simulink model "debugcurrentloop"  (R2024a)
settings: Solver=VariableStepAuto  StartTime=0.0  StopTime=5  RelTol=1e-3
model workspace (MAT data in the model file):
  Frequency_175 = 0
  TargetFrequency_175 = 2100000000
  uniqueStringPll_175 = '53_5733'
undefined symbols (not defined in the file): DiscIntNeverNeededParam
libraries: simulink x6, mcbcontrolslib x6, slpidlib x1, mcbplantlib x1, autolibpmsmexterior x1
settings Model: Creator=wsl  LastModifiedBy=wsl

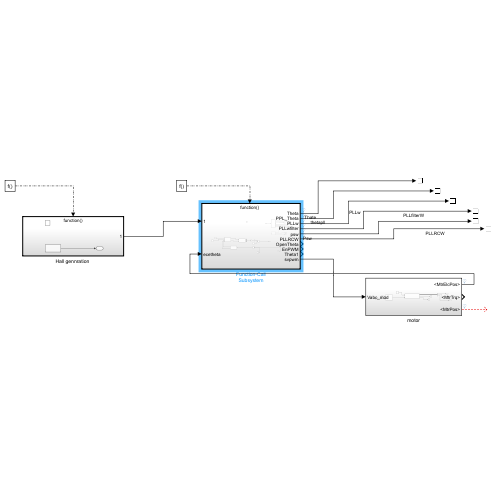
[thumbnail: Simulink's stored preview of the top-level diagram]
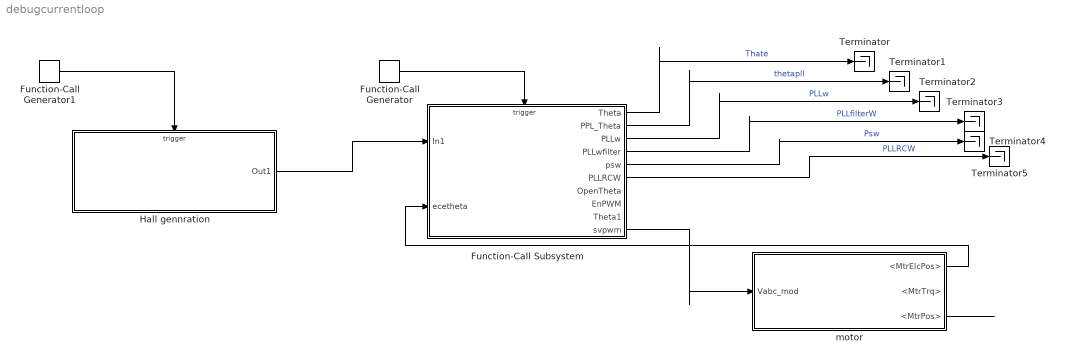
== system debugcurrentloop ==
  Function-Call Generator : simulink/Ports & Subsystems/Function-Call Generator  sample_time=1e-4  numberOfIterations=1  DisallowWideOutput=off
  Function-Call Generator1 : simulink/Ports & Subsystems/Function-Call Generator  sample_time=1/48  numberOfIterations=1  DisallowWideOutput=off
  Function-Call Subsystem : Subsystem  TreatAsAtomicUnit=on
  "Hall gennration " : Subsystem  TreatAsAtomicUnit=on
  Terminator{,1..5} (6 alike) : Terminator
  motor : Subsystem
  wires:
  Function-Call Generator/1 -> Function-Call Subsystem/Trigger
  Function-Call Generator1/1 -> "Hall gennration "/Trigger
  "Hall gennration "/1(Out1) -> Function-Call Subsystem/1(In1)
  Function-Call Subsystem/1(Theta) -> Terminator/1  "Thate"
  Function-Call Subsystem/2(PPL_Theta) -> Terminator1/1  "thetapll"
  Function-Call Subsystem/3(PLLw) -> Terminator2/1  "PLLw"
  Function-Call Subsystem/4(PLLwfilter) -> Terminator3/1  "PLLfilterW"
  Function-Call Subsystem/6(PLLRCW) -> Terminator5/1  "PLLRCW"
  Function-Call Subsystem/5(psw) -> Terminator4/1  "Psw"
  Function-Call Subsystem/10(svpwm) -> motor/1(Vabc_mod)
  motor/1(<MtrElcPos>) -> Function-Call Subsystem/2(ecetheta)
  motor/3(<MtrPos>) -> ?

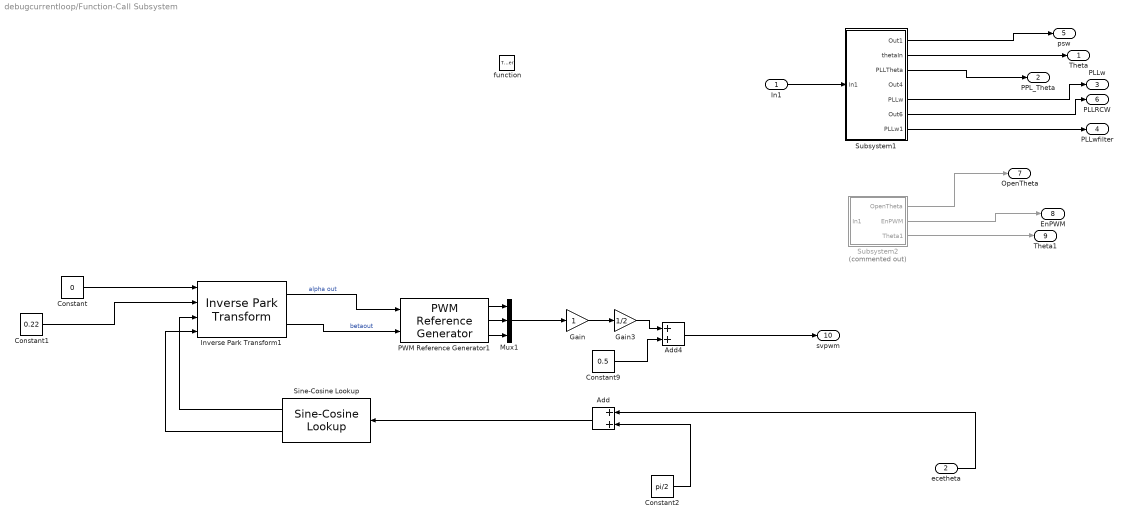
== system debugcurrentloop/Function-Call Subsystem ==
  In1 : Inport
  ecetheta : Inport  Port=2
  function : TriggerPort  TriggerType=function-call  VariantControl=(inherit)
  Add : Sum
  Add4 : Sum
  Constant : Constant  Value=0
  Constant1 : Constant  Value=0.22
  Constant2 : Constant  Value=pi/2
  Constant9 : Constant  Value=0.5
  Gain : Gain
  Gain3 : Gain  Gain=1/2
  Inverse Park Transform1 : mcbcontrolslib/Inverse Park Transform  PhaseInput=Two inputs  AxisAlignment=D-axis  ThetaInput=Sine and Cosine electrical position  AngleInput=Radians  N_points=1024
      settings: LibrarySourceBlock=mcblib/Controls/Math Transforms/Inverse Park Transform
  Mux1 : Mux  Inputs=3
  PWM Reference Generator1 : mcbcontrolslib/PWM Reference Generator  inSignal=Valphabeta  modType=SVM: space vector modulation
      settings: LibrarySourceBlock=mcblib/Controls/Math Transforms/PWM Reference Generator
  Sine-Cosine Lookup : mcbcontrolslib/Sine-Cosine Lookup  AngleInput=Radians  N_points=1024  DatatypeInput=Inherit from input  Datatype=single
      settings: LibrarySourceBlock=mcblib/Controls/Math Transforms/Sine-Cosine Lookup
  Subsystem1 : Subsystem
  Subsystem2 : Subsystem  Commented=on
  Theta : Outport
  PPL_Theta : Outport  Port=2
  PLLw : Outport  Port=3
  PLLwfilter : Outport  Port=4
  psw : Outport  Port=5
  PLLRCW : Outport  Port=6
  OpenTheta : Outport  Port=7
  EnPWM : Outport  Port=8
  Theta1 : Outport  Port=9
  svpwm : Outport  Port=10
  wires:
  In1/1 -> Subsystem1/1(In1)
  Subsystem1/1(Out1) -> psw/1
  Subsystem1/2(thetaIn) -> Theta/1
  Subsystem1/3(PLLTheta) -> PPL_Theta/1
  Subsystem1/5(PLLw) -> PLLw/1
  Subsystem1/6(Out6) -> PLLRCW/1
  Subsystem1/7(PLLw1) -> PLLwfilter/1
  Subsystem2/1(OpenTheta) -> OpenTheta/1
  Subsystem2/2(EnPWM) -> EnPWM/1
  Subsystem2/3(Theta1) -> Theta1/1
  Inverse Park Transform1/1 -> PWM Reference Generator1/1  "alpha out"
  Constant9/1 -> Add4/2
  Gain3/1 -> Add4/1
  Gain/1 -> Gain3/1
  PWM Reference Generator1/2 -> Mux1/2
  Inverse Park Transform1/2 -> PWM Reference Generator1/2  "betaout"
  PWM Reference Generator1/1 -> Mux1/1
  Add4/1 -> svpwm/1
  PWM Reference Generator1/3 -> Mux1/3
  Mux1/1 -> Gain/1
  Sine-Cosine Lookup/1 -> Inverse Park Transform1/3
  Sine-Cosine Lookup/2 -> Inverse Park Transform1/4
  Constant/1 -> Inverse Park Transform1/1
  Constant1/1 -> Inverse Park Transform1/2
  ecetheta/1 -> Add/1
  Constant2/1 -> Add/2
  Add/1 -> Sine-Cosine Lookup/1

== system debugcurrentloop/Hall gennration  ==
  function : TriggerPort  TriggerType=function-call  VariantControl=(inherit)
  Repeating Sequence Stair1 : simulink/Sources/Repeating Sequence Stair  OutValues=[1 5 4 6 2 3].'  tsamp=-1  OutMin=[]  OutMax=[]  OutDataTypeStr=double  OutputDataTypeScalingMode=double  OutDataType=fixdt(0,8)  ConRadixGroup=Best Precision: Vector-wise  OutScaling=2^-12
  Out1 : Outport
  wires:
  Repeating Sequence Stair1/1 -> Out1/1

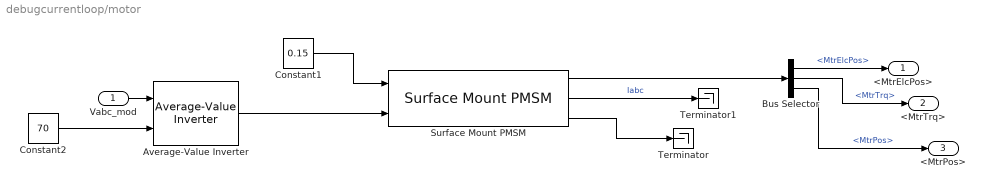
== system debugcurrentloop/motor ==
  Vabc_mod : Inport
  Average-Value Inverter : mcbplantlib/Average-Value Inverter
  Bus Selector : BusSelector  OutputSignals=MtrElcPos,MtrTrq,MtrPos
  Constant1 : Constant  Value=0.15
  Constant2 : Constant  Value=70
  Surface Mount PMSM : autolibpmsmexterior/Surface Mount PMSM  port_config=Torque  sim_type=Discrete  Ts=5e-6  P=2  Rs=8.85  Ldq_=28e-3  KConstText=Back-emf constant (Ke):  lambda_pm=0.2205  Ke=29  Kt=1.323  mechanical=[0.0027, 4.924e-4, 0]  idq0=[0 0]  theta_init=0  omega_init=0  KConst=0.2205  lambda_pm_calc=0.079943  RefBlkName='autolibpmsmexterior/Surface Mount PMSM'  aMode=5  Ldq="[0.0017      0.0017]"
  Terminator : Terminator
  Terminator1 : Terminator
  <MtrElcPos> : Outport
  <MtrTrq> : Outport  Port=2
  <MtrPos> : Outport  Port=3
  wires:
  Surface Mount PMSM/3 -> Terminator/1
  Constant2/1 -> Average-Value Inverter/2
  Vabc_mod/1 -> Average-Value Inverter/1
  Average-Value Inverter/1 -> Surface Mount PMSM/2
  Constant1/1 -> Surface Mount PMSM/1
  Surface Mount PMSM/2 -> Terminator1/1  "Iabc"
  Surface Mount PMSM/1 -> Bus Selector/1
  Bus Selector/1 -> <MtrElcPos>/1  "<MtrElcPos>"
  Bus Selector/2 -> <MtrTrq>/1  "<MtrTrq>"
  Bus Selector/3 -> <MtrPos>/1  "<MtrPos>"

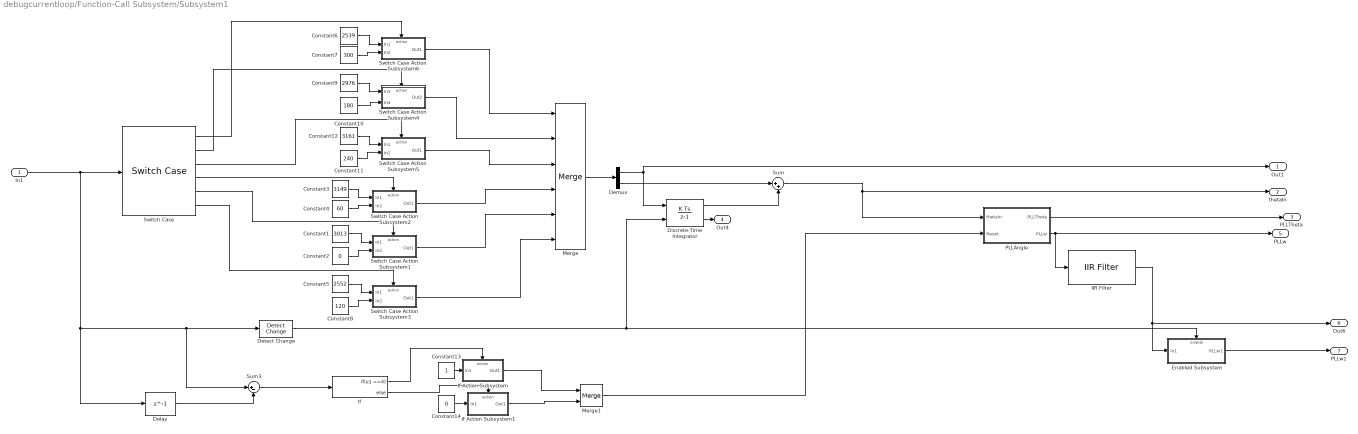
== system debugcurrentloop/Function-Call Subsystem/Subsystem1 ==
  In1 : Inport
  Constant1 : Constant  Value=3013
  Constant10 : Constant  Value=180
  Constant11 : Constant  Value=240
  Constant12 : Constant  Value=3161
  Constant13 : Constant  OutDataTypeStr=boolean
  Constant14 : Constant  Value=0  OutDataTypeStr=boolean
  Constant2 : Constant  Value=0
  Constant3 : Constant  Value=3149
  Constant4 : Constant  Value=60
  Constant5 : Constant  Value=2552
  Constant6 : Constant  Value=2539
  Constant7 : Constant  Value=300
  Constant8 : Constant  Value=120
  Constant9 : Constant  Value=2976
  Delay : Delay  DelayLength=1  InitialCondition=0  UseCircularBuffer=on
  Demux : Demux  Outputs=2
  Detect Change : simulink/Logic and Bit Operations/Detect Change  vinit=0  OutDataTypeStr=boolean
  Discrete-Time Integrator : DiscreteIntegrator  ExternalReset=rising  SampleTime=-1  LimitOutput=on  UpperSaturationLimit=60  LowerSaturationLimit=-60  ShowSaturationPort=on  ICPrevOutput=DiscIntNeverNeededParam  ICPrevScaledInput=DiscIntNeverNeededParam
  Enabled Subsystem : Subsystem  TreatAsAtomicUnit=on
  IIR Filter : mcbcontrolslib/IIR Filter  VariantControl=Low Pass Filter  VariantSelect=Low-pass  FilterConstantInputType=Specify via dialog  Filter_constant=0.01  advancedSettings=on  Ts=1e-4  cutOff_freq=16.0763
      settings: LibrarySourceBlock=mcbhdllib/Signal Management/IIR Filter
  If : If  IfExpression=u1 ==4
  If Action Subsystem : Subsystem  TreatAsAtomicUnit=on
  If Action Subsystem1 : Subsystem  TreatAsAtomicUnit=on
  Merge : Merge  Inputs=6
  Merge1 : Merge
  PLLAngle : Subsystem
  Sum : Sum  Inputs=|++
  Sum3 : Sum  Inputs=|+-
  Switch Case : SwitchCase  CaseConditions={1,2,3,4,5,6}  ShowDefaultCase=off
  Switch Case Action Subsystem1 : Subsystem  TreatAsAtomicUnit=on
  Switch Case Action Subsystem2 : Subsystem  TreatAsAtomicUnit=on
  Switch Case Action Subsystem3 : Subsystem  TreatAsAtomicUnit=on
  Switch Case Action Subsystem4 : Subsystem  TreatAsAtomicUnit=on
  Switch Case Action Subsystem5 : Subsystem  TreatAsAtomicUnit=on
  Switch Case Action Subsystem6 : Subsystem  TreatAsAtomicUnit=on
  Out1 : Outport
  thetaIn : Outport  Port=2
  PLLTheta : Outport  Port=3
  Out4 : Outport  Port=4
  PLLw : Outport  Port=5
  Out6 : Outport  Port=6
  PLLw1 : Outport  Port=7
  wires:
  Constant6/1 -> Switch Case Action Subsystem6/1(In1)
  Constant4/1 -> Switch Case Action Subsystem2/2(In2)
  Merge/1 -> Demux/1
  Switch Case/6 -> Switch Case Action Subsystem3/Action
  Constant8/1 -> Switch Case Action Subsystem3/2(In2)
  Switch Case/5 -> Switch Case Action Subsystem1/Action
  Switch Case Action Subsystem1/1(Out1) -> Merge/5
  Constant10/1 -> Switch Case Action Subsystem4/2(In4)
  Switch Case Action Subsystem6/1(Out1) -> Merge/1
  Demux/1 -> Out1/1, Discrete-Time Integrator/1
  Constant12/1 -> Switch Case Action Subsystem5/1(In1)
  Constant1/1 -> Switch Case Action Subsystem1/1(In1)
  Constant11/1 -> Switch Case Action Subsystem5/2(In2)
  Constant2/1 -> Switch Case Action Subsystem1/2(In2)
  Demux/2 -> Sum/1
  Constant9/1 -> Switch Case Action Subsystem4/1(In3)
  In1/1 -> Delay/1, Sum3/1, Detect Change/1, Switch Case/1
  Discrete-Time Integrator/2 -> Out4/1
  Switch Case/1 -> Switch Case Action Subsystem6/Action
  Constant7/1 -> Switch Case Action Subsystem6/2(In2)
  Switch Case/3 -> Switch Case Action Subsystem5/Action
  If Action Subsystem/1(Out1) -> Merge1/1
  Detect Change/1 -> Enabled Subsystem/Enable, Discrete-Time Integrator/2
  Constant3/1 -> Switch Case Action Subsystem2/1(In1)
  Constant13/1 -> If Action Subsystem/1(In1)
  Switch Case/2 -> Switch Case Action Subsystem4/Action
  Enabled Subsystem/1(PLLw1) -> PLLw1/1
  Switch Case/4 -> Switch Case Action Subsystem2/Action
  Switch Case Action Subsystem5/1(Out1) -> Merge/3
  PLLAngle/2(PLLw) -> PLLw/1, IIR Filter/1
  If/2 -> If Action Subsystem1/Action
  Constant5/1 -> Switch Case Action Subsystem3/1(In1)
  Sum3/1 -> If/1
  IIR Filter/1 -> Out6/1, Enabled Subsystem/1(In1)
  Sum/1 -> thetaIn/1, PLLAngle/1(thetaIn)
  If Action Subsystem1/1(Out1) -> Merge1/2
  Delay/1 -> Sum3/2
  Switch Case Action Subsystem3/1(Out1) -> Merge/6
  Switch Case Action Subsystem4/1(Out2) -> Merge/2
  Constant14/1 -> If Action Subsystem1/1(In1)
  Merge1/1 -> PLLAngle/2(Reset)
  PLLAngle/1(PLLTheta) -> PLLTheta/1
  If/1 -> If Action Subsystem/Action
  Switch Case Action Subsystem2/1(Out1) -> Merge/4
  Discrete-Time Integrator/1 -> Sum/2

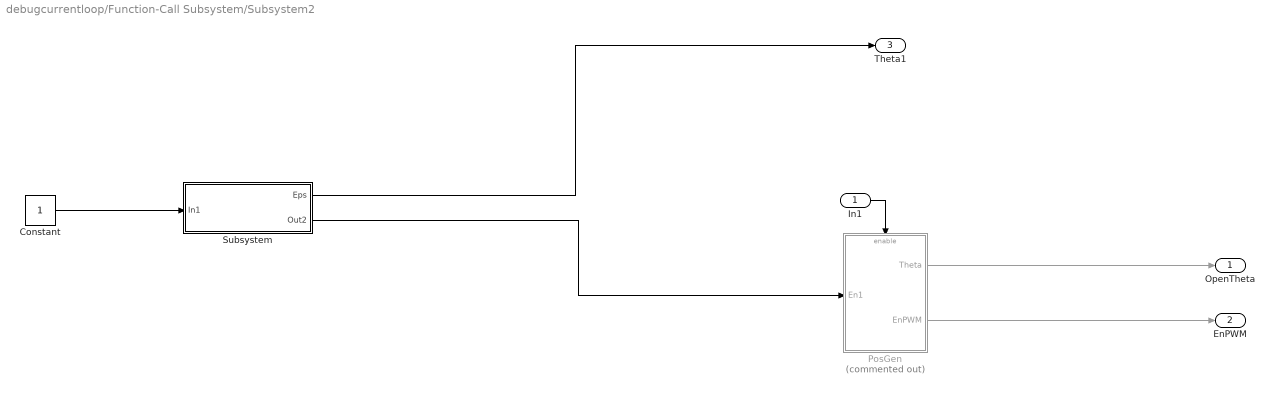
== system debugcurrentloop/Function-Call Subsystem/Subsystem2 ==
  In1 : Inport
  Constant : Constant
  PosGen : Subsystem  Commented=on
  Subsystem : Subsystem
  OpenTheta : Outport
  EnPWM : Outport  Port=2
  Theta1 : Outport  Port=3
  wires:
  PosGen/1(Theta) -> OpenTheta/1
  PosGen/2(EnPWM) -> EnPWM/1
  Constant/1 -> Subsystem/1(In1)
  Subsystem/2(Out2) -> PosGen/1(En1)
  Subsystem/1(Eps) -> Theta1/1
  In1/1 -> PosGen/Enable

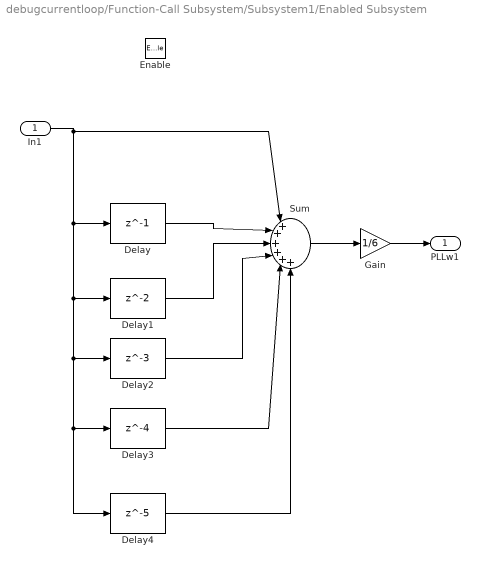
== system debugcurrentloop/Function-Call Subsystem/Subsystem1/Enabled Subsystem ==
  In1 : Inport
  Enable : EnablePort
  Delay : Delay  DelayLength=1  InitialCondition=0  UseCircularBuffer=on
  Delay1 : Delay  InitialCondition=0  UseCircularBuffer=on
  Delay2 : Delay  DelayLength=3  InitialCondition=0  UseCircularBuffer=on
  Delay3 : Delay  DelayLength=4  InitialCondition=0  UseCircularBuffer=on
  Delay4 : Delay  DelayLength=5  InitialCondition=0  UseCircularBuffer=on
  Gain : Gain  Gain=1/6
  Sum : Sum  Inputs=|++++++
  PLLw1 : Outport
  wires:
  In1/1 -> Delay4/1, Delay3/1, Delay2/1, Delay1/1, Delay/1, Sum/1
  Delay/1 -> Sum/2
  Delay1/1 -> Sum/3
  Sum/1 -> Gain/1
  Gain/1 -> PLLw1/1
  Delay2/1 -> Sum/4
  Delay3/1 -> Sum/5
  Delay4/1 -> Sum/6

== system debugcurrentloop/Function-Call Subsystem/Subsystem1/If Action Subsystem ==
  In1 : Inport
  Action Port : ActionPort  ActionPortLabel=if(u1 ==4)
  Out1 : Outport
  wires:
  In1/1 -> Out1/1

== system debugcurrentloop/Function-Call Subsystem/Subsystem1/If Action Subsystem1 ==
  In1 : Inport
  Action Port : ActionPort  ActionPortLabel=else
  Out1 : Outport
  wires:
  In1/1 -> Out1/1

== system debugcurrentloop/Function-Call Subsystem/Subsystem1/PLLAngle ==
  thetaIn : Inport
  Reset : Inport  Port=2
  Discrete-Time Integrator1 : DiscreteIntegrator  ExternalReset=rising  SampleTime=-1  LimitOutput=on  UpperSaturationLimit=360  LowerSaturationLimit=0  IgnoreLimit=on  ICPrevOutput=DiscIntNeverNeededParam  ICPrevScaledInput=DiscIntNeverNeededParam
  PID Controller : slpidlib/PID Controller  Controller=PI  Form=Parallel  TimeDomain=Discrete-time  UseExternalTs=off  SampleTime=-1  IntegratorMethod=Forward Euler  FilterMethod=Forward Euler  ControllerParametersSource=internal  P=530  I=0.28  UseKiTs=off  D=0  UseExternalDerivativeSource=off  N=100  UseFilter=on  TunerSelectOption=Transfer Function Based (PID Tuner App)  InitialConditionSource=internal  InitialConditionForIntegrator=0  InitialConditionForFilter=0  DifferentiatorICPrevScaledInput=0  ExternalReset=none  TrackingMode=off  Kt=1  LimitOutput=off  SatLimitsSource=internal  UpperSaturationLimit=inf  LowerSaturationLimit=-inf  LinearizeAsGain=on  AntiWindupMode=none  Kb=1  LimitIntegrator=off  UpperIntegratorSaturationLimit=inf  LowerIntegratorSaturationLimit=-inf  POutMin=[]  POutMax=[]  IOutMin=[]  IOutMax=[]  DOutMin=[]  DOutMax=[]  NOutMin=[]  NOutMax=[]  SumOutMin=[]  SumOutMax=[]  SaturationOutMin=[]  SaturationOutMax=[]  PParamMin=[]  PParamMax=[]  IParamMin=[]  IParamMax=[]  DParamMin=[]  DParamMax=[]  NParamMin=[]  NParamMax=[]  KbParamMin=[]  KbParamMax=[]  KtParamMin=[]  KtParamMax=[]  KbOutMin=[]  KbOutMax=[]  KtOutMin=[]  KtOutMax=[]  IntegratorOutMin=[]  IntegratorOutMax=[]  FilterOutMin=[]  FilterOutMax=[]  SumI1OutMin=[]  SumI1OutMax=[]  SumI2OutMin=[]  SumI2OutMax=[]  SumI3OutMin=[]  SumI3OutMax=[]  SumI4OutMin=[]  SumI4OutMax=[]  SumDOutMin=[]  SumDOutMax=[]  DifferentiatorOutMin=[]  DifferentiatorOutMax=[]  FilterDiffOutCoefMin=[]  FilterDiffOutCoefMax=[]  ReciprocalOutMin=[]  ReciprocalOutMax=[]  SumDenOutMin=[]  SumDenOutMax=[]  SumNumOutMin=[]  SumNumOutMax=[]  DivideOutMin=[]  DivideOutMax=[]  UdiffTsProdOutMin=[]  UdiffTsProdOutMax=[]  NTsProdOutMin=[]  NTsProdOutMax=[]  UintegralTsProdOutMin=[]  UintegralTsProdOutMax=[]  UngainTsProdOutMin=[]  UngainTsProdOutMax=[]  ClampingZeroOutDataTypeStr=Inherit: Inherit via back propagation  ClampingZeroOutMin=[]  ClampingZeroOutMax=[]  FilterDenConstantOutDataTypeStr=Inherit: Inherit via back propagation  FilterDenConstantOutMin=[]  FilterDenConstantOutMax=[]  PCopyOutDataTypeStr=Inherit: Inherit via back propagation  PCopyOutMin=[]  PCopyOutMax=[]  NCopyOutDataTypeStr=Inherit: Inherit via back propagation  NCopyOutMin=[]  NCopyOutMax=[]  IntegratorContinuousStateAttributes=''  IntegratorStateMustResolveToSignalObject=off  IntegratorRTWStateStorageClass=Auto  FilterContinuousStateAttributes=''  FilterStateMustResolveToSignalObject=off  FilterRTWStateStorageClass=Auto  ParallelPVariant=InternalParameters  IdealPVariant=Disabled  IVariant=InternalParameters  DVariant=Disabled  IntegratorVariant=Discrete  SatVariant=Disabled  AWVariant=Passthrough  PCopyVariant=Disabled  TRVariant=Disabled  FdbkBlocksVariant=Forward  IdealPFdbkVariant=Disabled  SatFdbkVariant=Disabled  DerivativeFilterVariant=Disabled  NVariant=Disabled  NCopyVariant=Disabled_SignalSpec  FilterICVariant=Disabled  IntegratorICVariant=InternalICs  ExternalResetVariant=Disabled  TRSumVariant=Passthrough  SumFdbkVariant=Disabled  SumVariant=Sum_PI  TsampFilterVariant=InternalTs  TsampNgainVariant=Passthrough  TsampIntegralVariant=Disabled_SignalSpec  ExternalSaturationOutDataTypeStr=Inherit: Same as second input  DerivativeSourceVariant=Disabled
  Sum1 : Sum  Inputs=|+-
  PLLTheta : Outport
  PLLw : Outport  Port=2
  wires:
  Sum1/1 -> PID Controller/1
  Discrete-Time Integrator1/1 -> PLLTheta/1, Sum1/2
  thetaIn/1 -> Sum1/1
  PID Controller/1 -> PLLw/1, Discrete-Time Integrator1/1
  Reset/1 -> Discrete-Time Integrator1/2

== system debugcurrentloop/Function-Call Subsystem/Subsystem1/Switch Case Action Subsystem1 ==
  In1 : Inport
  In2 : Inport  Port=2
  Action Port : ActionPort  ActionPortLabel=case [ 5 ]:
  Mux : Mux  Inputs=2
  Out1 : Outport
  wires:
  In1/1 -> Mux/1
  In2/1 -> Mux/2
  Mux/1 -> Out1/1

== system debugcurrentloop/Function-Call Subsystem/Subsystem1/Switch Case Action Subsystem2 ==
  In1 : Inport
  In2 : Inport  Port=2
  Action Port : ActionPort  ActionPortLabel=case [ 4 ]:
  Mux : Mux  Inputs=2
  Out1 : Outport
  wires:
  In1/1 -> Mux/1
  In2/1 -> Mux/2
  Mux/1 -> Out1/1

== system debugcurrentloop/Function-Call Subsystem/Subsystem1/Switch Case Action Subsystem3 ==
  In1 : Inport
  In2 : Inport  Port=2
  Action Port : ActionPort  ActionPortLabel=case [ 6 ]:
  Mux : Mux  Inputs=2
  Out1 : Outport
  wires:
  In1/1 -> Mux/1
  In2/1 -> Mux/2
  Mux/1 -> Out1/1

== system debugcurrentloop/Function-Call Subsystem/Subsystem1/Switch Case Action Subsystem4 ==
  In3 : Inport
  In4 : Inport  Port=2
  Action Port : ActionPort  ActionPortLabel=case [ 2 ]:
  Mux : Mux  Inputs=2
  Out2 : Outport
  wires:
  Mux/1 -> Out2/1
  In3/1 -> Mux/1
  In4/1 -> Mux/2

== system debugcurrentloop/Function-Call Subsystem/Subsystem1/Switch Case Action Subsystem5 ==
  In1 : Inport
  In2 : Inport  Port=2
  Action Port : ActionPort  ActionPortLabel=case [ 3 ]:
  Mux : Mux  Inputs=2
  Out1 : Outport
  wires:
  In1/1 -> Mux/1
  In2/1 -> Mux/2
  Mux/1 -> Out1/1

== system debugcurrentloop/Function-Call Subsystem/Subsystem1/Switch Case Action Subsystem6 ==
  In1 : Inport
  In2 : Inport  Port=2
  Action Port : ActionPort  ActionPortLabel=case [ 1 ]:
  Mux : Mux  Inputs=2
  Out1 : Outport
  wires:
  Mux/1 -> Out1/1
  In1/1 -> Mux/1
  In2/1 -> Mux/2

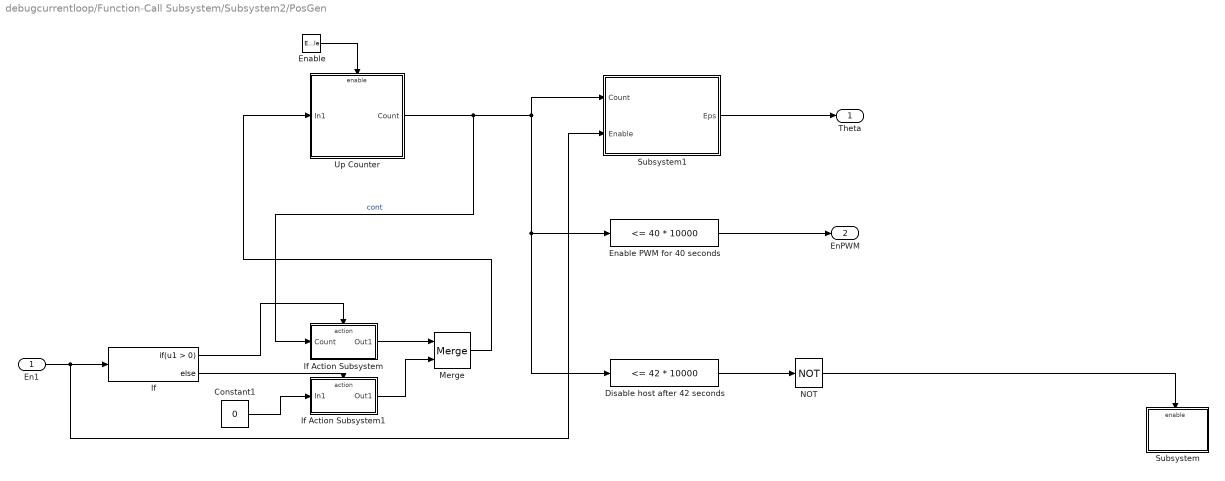
== system debugcurrentloop/Function-Call Subsystem/Subsystem2/PosGen ==
  En1 : Inport
  Enable : EnablePort  StatesWhenEnabling=reset  ShowOutputPort=on
  Constant1 : Constant  Value=0  OutDataTypeStr=uint32
  Disable host after 42 seconds : simulink/Logic and Bit Operations/Compare To Constant  relop=<=  const=42 * 10000  OutDataTypeStr=boolean
  Enable PWM for 40 seconds : simulink/Logic and Bit Operations/Compare To Constant  relop=<=  const=40 * 10000  OutDataTypeStr=boolean
  If : If
  If Action Subsystem : Subsystem  TreatAsAtomicUnit=on
  If Action Subsystem1 : Subsystem  TreatAsAtomicUnit=on
  Merge : Merge
  NOT : Logic  Operator=NOT  IconShape=distinctive  AllPortsSameDT=off  OutDataTypeStr=boolean
  Subsystem : Subsystem
  Subsystem1 : Subsystem
  Up Counter : Subsystem
  Theta : Outport
  EnPWM : Outport  Port=2  OutputWhenDisabled=reset  InitialOutput=0  VectorParamsAs1DForOutWhenUnconnected=off
  wires:
  Subsystem1/1(Eps) -> Theta/1
  Enable/1 -> Up Counter/Enable
  NOT/1 -> Subsystem/Enable
  Enable PWM for 40 seconds/1 -> EnPWM/1
  Disable host after 42 seconds/1 -> NOT/1
  Merge/1 -> Up Counter/1(In1)
  If/1 -> If Action Subsystem/Action
  If Action Subsystem/1(Out1) -> Merge/1
  Up Counter/1(Count) -> If Action Subsystem/1(Count), Disable host after 42 seconds/1, Enable PWM for 40 seconds/1, Subsystem1/1(Count)  "cont"
  If/2 -> If Action Subsystem1/Action
  If Action Subsystem1/1(Out1) -> Merge/2
  Constant1/1 -> If Action Subsystem1/1(In1)
  En1/1 -> Subsystem1/2(Enable), If/1

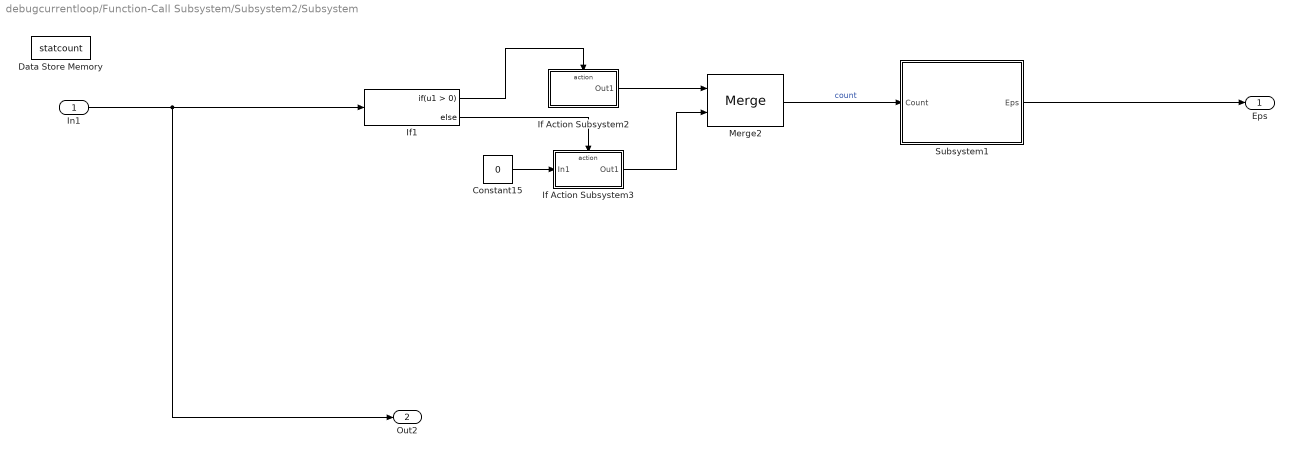
== system debugcurrentloop/Function-Call Subsystem/Subsystem2/Subsystem ==
  In1 : Inport
  Constant15 : Constant  Value=0  OutDataTypeStr=uint32
  Data Store Memory : DataStoreMemory  DataStoreName=statcount  WriteAfterWriteMsg=warning  ShowAdditionalParam=off
  If Action Subsystem2 : Subsystem  TreatAsAtomicUnit=on
  If Action Subsystem3 : Subsystem  TreatAsAtomicUnit=on
  If1 : If
  Merge2 : Merge
  Subsystem1 : Subsystem
  Eps : Outport
  Out2 : Outport  Port=2
  wires:
  If1/2 -> If Action Subsystem3/Action
  In1/1 -> Out2/1, If1/1
  Subsystem1/1(Eps) -> Eps/1
  If1/1 -> If Action Subsystem2/Action
  If Action Subsystem3/1(Out1) -> Merge2/2
  Constant15/1 -> If Action Subsystem3/1(In1)
  If Action Subsystem2/1(Out1) -> Merge2/1
  Merge2/1 -> Subsystem1/1(Count)  "count"

== system debugcurrentloop/Function-Call Subsystem/Subsystem2/PosGen/If Action Subsystem ==
  Count : Inport
  Action Port : ActionPort  ActionPortLabel=if(u1 > 0)
  Out1 : Outport
  wires:
  Count/1 -> Out1/1

== system debugcurrentloop/Function-Call Subsystem/Subsystem2/PosGen/If Action Subsystem1 ==
  In1 : Inport
  Action Port : ActionPort  ActionPortLabel=else
  Out1 : Outport
  wires:
  In1/1 -> Out1/1

== system debugcurrentloop/Function-Call Subsystem/Subsystem2/PosGen/Subsystem ==
  Enable : EnablePort

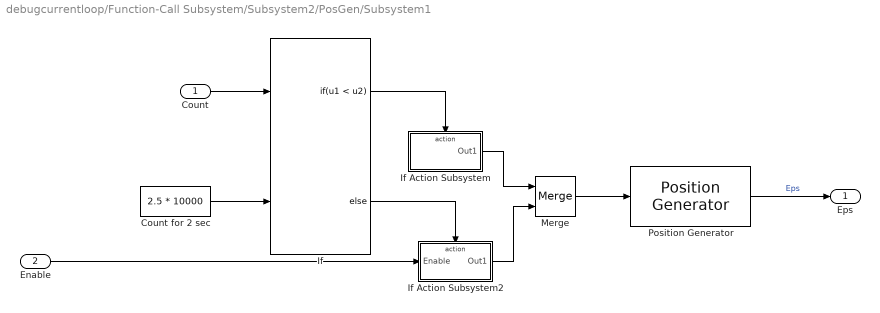
== system debugcurrentloop/Function-Call Subsystem/Subsystem2/PosGen/Subsystem1 ==
  Count : Inport
  Enable : Inport  Port=2
  Count for 2 sec : Constant  Value=2.5 * 10000  OutDataTypeStr=uint32  SampleTime=-1
  If : If  NumInputs=2  IfExpression=u1 < u2
  If Action Subsystem : Subsystem  TreatAsAtomicUnit=on
  If Action Subsystem2 : Subsystem  TreatAsAtomicUnit=on
  Merge : Merge
  Position Generator : mcbcontrolslib/Position Generator  AngleOutput=Per-unit  ExternalReset=none  Offset=0
  Eps : Outport
  wires:
  If Action Subsystem/1(Out1) -> Merge/1
  If/1 -> If Action Subsystem/Action
  If Action Subsystem2/1(Out1) -> Merge/2
  Position Generator/1 -> Eps/1  "Eps"
  Count/1 -> If/1
  Merge/1 -> Position Generator/1
  If/2 -> If Action Subsystem2/Action
  Count for 2 sec/1 -> If/2
  Enable/1 -> If Action Subsystem2/1(Enable)

== system debugcurrentloop/Function-Call Subsystem/Subsystem2/PosGen/Up Counter ==
  In1 : Inport
  Enable : EnablePort  StatesWhenEnabling=reset
  Add1 : Sum  SaturateOnIntegerOverflow=on
  Constant : Constant  OutDataTypeStr=uint32
  Delay : Delay  DelayLength=1
  Count : Outport  OutputWhenDisabled=reset  InitialOutput=0
  wires:
  Add1/1 -> Count/1
  Constant/1 -> Add1/1
  Delay/1 -> Add1/2
  In1/1 -> Delay/1

== system debugcurrentloop/Function-Call Subsystem/Subsystem2/Subsystem/If Action Subsystem2 ==
  Action Port : ActionPort  ActionPortLabel=if(u1 > 0)
  Add1 : Sum  SaturateOnIntegerOverflow=on
  Constant : Constant  OutDataTypeStr=uint32
  Data Store Read : DataStoreRead  DataStoreName=statcount  IndexOptions=Index vector (dialog)  Indices=1  OutputSizes=1
  Data Store Write : DataStoreWrite  DataStoreName=statcount  IndexOptions=Index vector (dialog)  Indices=1  OutputSizes=1
  Out1 : Outport
  wires:
  Add1/1 -> Data Store Write/1, Out1/1
  Data Store Read/1 -> Add1/2
  Constant/1 -> Add1/1

== system debugcurrentloop/Function-Call Subsystem/Subsystem2/Subsystem/If Action Subsystem3 ==
  In1 : Inport
  Action Port : ActionPort  ActionPortLabel=else
  Data Store Write : DataStoreWrite  DataStoreName=statcount  IndexOptions=Index vector (dialog)  Indices=1  OutputSizes=1
  Out1 : Outport
  wires:
  In1/1 -> Data Store Write/1, Out1/1

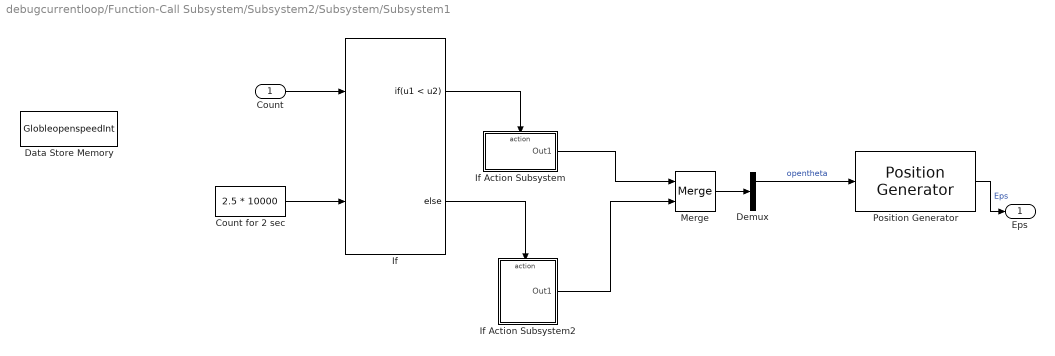
== system debugcurrentloop/Function-Call Subsystem/Subsystem2/Subsystem/Subsystem1 ==
  Count : Inport
  Count for 2 sec : Constant  Value=2.5 * 10000  OutDataTypeStr=uint32  SampleTime=-1
  Data Store Memory : DataStoreMemory  DataStoreName=GlobleopenspeedInt  WriteAfterWriteMsg=warning  ShowAdditionalParam=off
  Demux : Demux  Outputs=2
  If : If  NumInputs=2  IfExpression=u1 < u2
  If Action Subsystem : Subsystem  TreatAsAtomicUnit=on
  If Action Subsystem2 : Subsystem  TreatAsAtomicUnit=on
  Merge : Merge
  Position Generator : mcbcontrolslib/Position Generator  AngleOutput=Per-unit  ExternalReset=none  Offset=0
  Eps : Outport
  wires:
  If Action Subsystem/1(Out1) -> Merge/1
  If/1 -> If Action Subsystem/Action
  If Action Subsystem2/1(Out1) -> Merge/2
  Position Generator/1 -> Eps/1  "Eps"
  Count/1 -> If/1
  If/2 -> If Action Subsystem2/Action
  Count for 2 sec/1 -> If/2
  Merge/1 -> Demux/1
  Demux/1 -> Position Generator/1  "opentheta"

== system debugcurrentloop/Function-Call Subsystem/Subsystem2/PosGen/Subsystem1/If Action Subsystem ==
  Action Port : ActionPort  ActionPortLabel=if(u1 < u2)
  Constant : Constant  Value=0  OutDataTypeStr=single
  Out1 : Outport
  wires:
  Constant/1 -> Out1/1

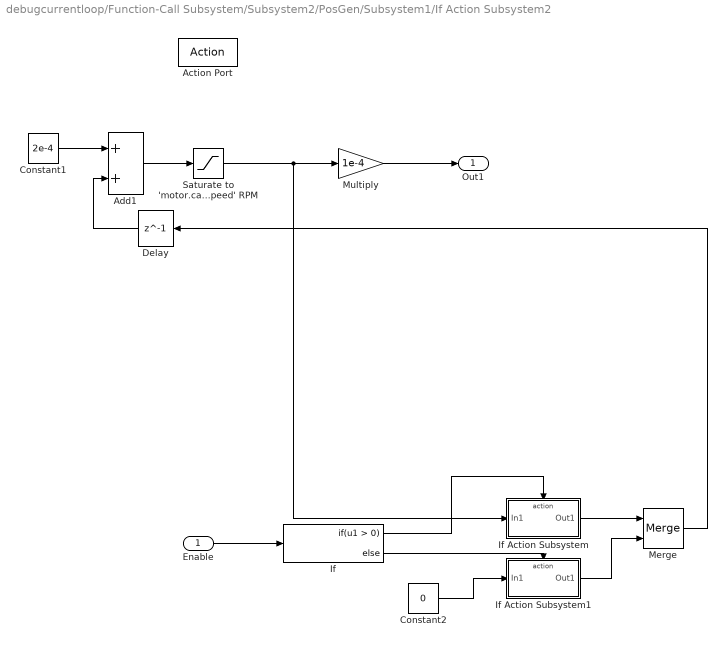
== system debugcurrentloop/Function-Call Subsystem/Subsystem2/PosGen/Subsystem1/If Action Subsystem2 ==
  Enable : Inport
  Action Port : ActionPort  ActionPortLabel=else
  Add1 : Sum
  Constant1 : Constant  Value=2e-4  VectorParams1D=off  OutDataTypeStr=single
  Constant2 : Constant  Value=0  OutDataTypeStr=single
  Delay : Delay  DelayLength=1
  If : If
  If Action Subsystem : Subsystem  TreatAsAtomicUnit=on
  If Action Subsystem1 : Subsystem  TreatAsAtomicUnit=on
  Merge : Merge
  Multiply : Gain  Gain=1e-4  OutDataTypeStr=Inherit: Same as input
  Saturate to 'motor.calibSpeed' RPM : Saturate  UpperLimit=2 *240/ 60  LowerLimit=0
  Out1 : Outport
  wires:
  Delay/1 -> Add1/2
  Constant1/1 -> Add1/1
  Multiply/1 -> Out1/1
  Add1/1 -> Saturate to 'motor.calibSpeed' RPM/1
  If/1 -> If Action Subsystem/Action
  If Action Subsystem/1(Out1) -> Merge/1
  Saturate to 'motor.calibSpeed' RPM/1 -> If Action Subsystem/1(In1), Multiply/1
  If/2 -> If Action Subsystem1/Action
  If Action Subsystem1/1(Out1) -> Merge/2
  Enable/1 -> If/1
  Constant2/1 -> If Action Subsystem1/1(In1)
  Merge/1 -> Delay/1

== system debugcurrentloop/Function-Call Subsystem/Subsystem2/Subsystem/Subsystem1/If Action Subsystem ==
  Action Port : ActionPort  ActionPortLabel=if(u1 < u2)
  Constant : Constant  Value=0  OutDataTypeStr=single
  Data Store Write : DataStoreWrite  DataStoreName=GlobleopenspeedInt  IndexOptions=Index vector (dialog)  Indices=1  OutputSizes=1
  Mux : Mux  Inputs=2
  Out1 : Outport
  wires:
  Constant/1 -> Data Store Write/1, Mux/2, Mux/1
  Mux/1 -> Out1/1

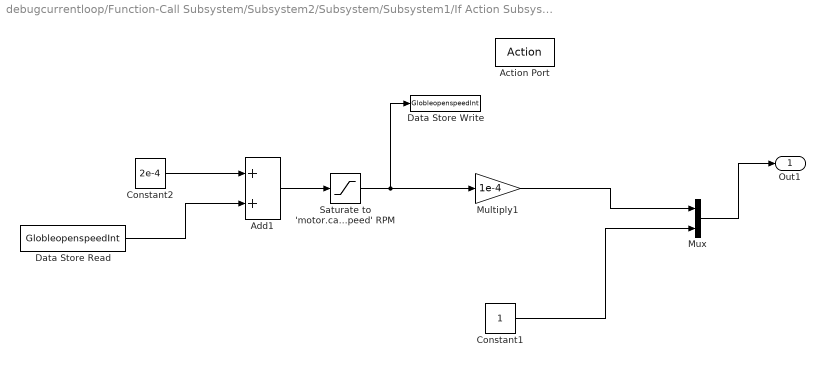
== system debugcurrentloop/Function-Call Subsystem/Subsystem2/Subsystem/Subsystem1/If Action Subsystem2 ==
  Action Port : ActionPort  ActionPortLabel=else
  Add1 : Sum
  Constant1 : Constant  VectorParams1D=off  OutDataTypeStr=single
  Constant2 : Constant  Value=2e-4  VectorParams1D=off  OutDataTypeStr=single
  Data Store Read : DataStoreRead  DataStoreName=GlobleopenspeedInt  IndexOptions=Index vector (dialog)  Indices=1  OutputSizes=1
  Data Store Write : DataStoreWrite  DataStoreName=GlobleopenspeedInt  IndexOptions=Index vector (dialog)  Indices=1  OutputSizes=1
  Multiply1 : Gain  Gain=1e-4  OutDataTypeStr=Inherit: Same as input
  Mux : Mux  Inputs=2
  Saturate to 'motor.calibSpeed' RPM : Saturate  UpperLimit=2 *240/ 60  LowerLimit=0
  Out1 : Outport
  wires:
  Constant1/1 -> Mux/2
  Mux/1 -> Out1/1
  Constant2/1 -> Add1/1
  Saturate to 'motor.calibSpeed' RPM/1 -> Data Store Write/1, Multiply1/1
  Data Store Read/1 -> Add1/2
  Add1/1 -> Saturate to 'motor.calibSpeed' RPM/1
  Multiply1/1 -> Mux/1

== system debugcurrentloop/Function-Call Subsystem/Subsystem2/PosGen/Subsystem1/If Action Subsystem2/If Action Subsystem ==
  In1 : Inport
  Action Port : ActionPort  ActionPortLabel=if(u1 > 0)
  Out1 : Outport
  wires:
  In1/1 -> Out1/1

== system debugcurrentloop/Function-Call Subsystem/Subsystem2/PosGen/Subsystem1/If Action Subsystem2/If Action Subsystem1 ==
  In1 : Inport
  Action Port : ActionPort  ActionPortLabel=else
  Out1 : Outport
  wires:
  In1/1 -> Out1/1
